simulink model "my_ODE_block"  (R2021a)
settings: Solver=VariableStepAuto  StartTime=0.0  StopTime=10.0  RelTol=1e-3
settings Model: Creator=jonathanbopp  LastModifiedBy=jonathanbopp

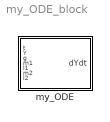
== system my_ODE_block ==
  my_ODE : MATLAB Function  TreatAsAtomicUnit=on

== matlab function my_ODE_block/my_ODE ==
  data: t input; dYdt output; Y input; g input; m1 input; l1 input; m2 input; l2 input
function dYdt = my_ODE(t,Y,g,m1,l1,m2,l2)
%#codegen

%    This function was generated by the Symbolic Math Toolbox version 8.7.
%    10-May-2021 19:37:08

t2 = Y(1);
t3 = Y(2);
t4 = Y(3);
t5 = Y(4);
t6 = sin(t2);
t7 = sin(t4);
t8 = t3.^2;
t9 = t5.^2;
t10 = -t4;
t11 = t2+t10;
t12 = cos(t11);
t13 = sin(t11);
t14 = t12.^2;
dYdt = [t3;-(g.*m1.*t6+g.*m2.*t6-g.*m2.*t7.*t12+l2.*m2.*t9.*t13+l1.*m2.*t8.*t12.*t13)./(l1.*m1+l1.*m2-l1.*m2.*t14);t5;(-g.*m1.*t7-g.*m2.*t7+g.*m1.*t6.*t12+g.*m2.*t6.*t12+l1.*m1.*t8.*t13+l1.*m2.*t8.*t13+l2.*m2.*t9.*t12.*t13)./(l2.*(m1+m2-m2.*t14))];
